simulink model "zynqRadioHWSWQPSKAD9361AD9364SL_interface"  (R2025a)
settings: Solver=FixedStepDiscrete  StartTime=0.0  StopTime=inf  RelTol=1e-3  EnableMultiTasking=on
PreLoadFcn:
  | HostIP = '192.168.3.1';
  | 
  | setTxBurstLength = 10000;
  | txtmsg = ['Zynq radio HW/SW Co-design QPSK']; % Use only printable characters
  | 
  | %------------------------------------------------------------------------------------------------------
  | 
  | if ~isequal(size(txtmsg),[1 31])
  |     error('txtmsg must contain 31 characters');
  | end
  | swTs = 0.02;
  | SamplesPerSymbol = 4;
  | Rsym = 1.92e6;
  | fs = Rsym*SamplesPerSymbol;
  | word = [txtmsg newline];
  | 
  | % The highest clock rate is 16 times the message character rate.
  | % As the message characters are fed at highest clock to FPGA
  | % repeat each character 16 times to maintain the message rate.
  | word = reshape(repmat(word,16,1),[],1);
  | repeatTimes = ceil(setTxBurstLength/length(word));
  | inpData = complex(repmat(uint8(word),repeatTimes,1));
  | inUseTxBurstLength = length(inpData);
InitFcn:
  | HostIP = '192.168.3.1';
  | 
  | setTxBurstLength = 10000;
  | txtmsg = ['Zynq radio HW/SW Co-design QPSK']; % Use only printable characters
  | 
  | %------------------------------------------------------------------------------------------------------
  | 
  | if ~isequal(size(txtmsg),[1 31])
  |     error('txtmsg must contain 31 characters');
  | end
  | swTs = 0.02;
  | SamplesPerSymbol = 4;
  | Rsym = 1.92e6;
  | fs = Rsym*SamplesPerSymbol;
  | word = [txtmsg newline];
  | 
  | % The highest clock rate is 16 times the message character rate.
  | % As the message characters are fed at highest clock to FPGA
  | % repeat each character 16 times to maintain the message rate.
  | word = reshape(repmat(word,16,1),[],1);
  | repeatTimes = ceil(setTxBurstLength/length(word));
  | inpData = complex(repmat(uint8(word),repeatTimes,1));
  | inUseTxBurstLength = length(inpData);
undefined symbols (not defined in the file or in its folder): AXI4, complex, Fs, ip, Lite
libraries: axiinterfacelib x10, zynqlib x3, xilinxsocad936xlib x2, axi_iio_lib x1, sdrzblksprivate x1
CloseFcn:
  | clear fs HostIP inpData inUseTxBurstLength ...
  |         repeatTimes Rsym SamplesPerSymbol ...
  |         setTxBurstLength swTs txtmsg word
settings Model: SimulationMode=accelerator  Creator=The MathWorks, Inc.  LastModifiedBy=The MathWorks, Inc.
settings SolverCC: AlgebraicLoopSolver=TrustRegion  PositivePriorityOrder=on  MaxZcPerStep=1.0
settings DataIOCC: ReturnWorkspaceOutputs=off
settings OptimizationCC: BlockReduction=off  ConditionallyExecuteInputs=off  EnhancedBackFolding=on  PassReuseOutputArgsAs=Individual arguments  ZeroExternalMemoryAtStartup=off  ZeroInternalMemoryAtStartup=off  MaxStackSize=64  OptimizeBlockOrder=speed  DifferentSizesBufferReuse=on  OptimizationCustomize=off  EfficientTunableParamExpr=on
settings DebuggingCC: AlgebraicLoopMsg=error  SingleTaskRateTransMsg=error  ParameterTunabilityLossMsg=error  UnconnectedInputMsg=warning  UnconnectedOutputMsg=warning  UnconnectedLineMsg=warning
settings HardwareCC: ProdBitPerPointer=32.0  ProdBitPerSizeT=32.0  ProdBitPerPtrDiffT=32.0  ProdLargestAtomicInteger=Long  ProdLargestAtomicFloat=Double  ProdWordSize=32.0  ProdLongLongMode=on  ProdHWDeviceType=ARM Compatible->ARM Cortex  TargetLargestAtomicInteger=Long  TargetLargestAtomicFloat=Double  TargetLongLongMode=on  TargetIntDivRoundTo=Zero  TargetEndianess=LittleEndian  TargetHWDeviceType=ARM Compatible->ARM Cortex
settings ModelReferenceCC: EnableRefExpFcnMdlSchedulingChecks=on  ModelReferenceNumInstancesAllowed=Single
settings SFSimCC: MATLABDynamicMemAlloc=off
settings RTWCC: SystemTargetFile=ert.tlc  HardwareBoard=Xilinx Zynq-7000 Based IIO Radio  TLCOptions="-aInlineSetEventsForThisBaseRateFcn=TLC_FALSE -aSuppressMultiTaskScheduler=TLC_FALSE  -aRateBasedStepFcn=0"  TemplateMakefile=ert_default_tmf  Toolchain=Linaro AArch32 Linux v6.3.1  GPUComputeCapability=3.5  DLArmComputeVersion=19.05  Description=Embedded Coder
settings CodeAppCC: ForceParamTrailComments=on  IgnoreCustomStorageClasses=off  OperatorAnnotations=on  SimulinkDataObjDesc=on  SFDataObjDesc=on  InsertBlockDesc=on
settings ERTTargetCC: ExtModeTransport=0.0  ExtModeStaticAlloc=off  ExtModeMexFile=ext_comm  ExtModeIntrfLevel=Level1  InlinedParameterPlacement=Hierarchical

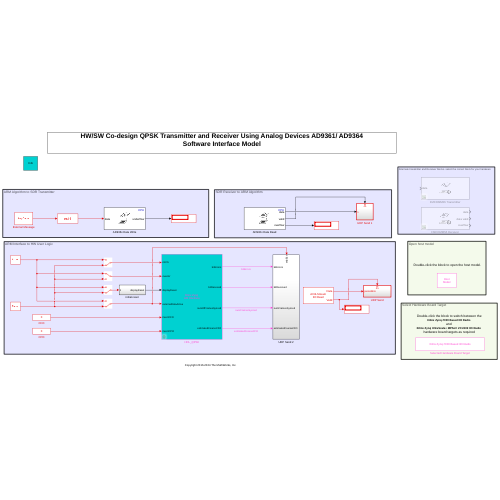
[thumbnail: Simulink's stored preview of the top-level diagram]
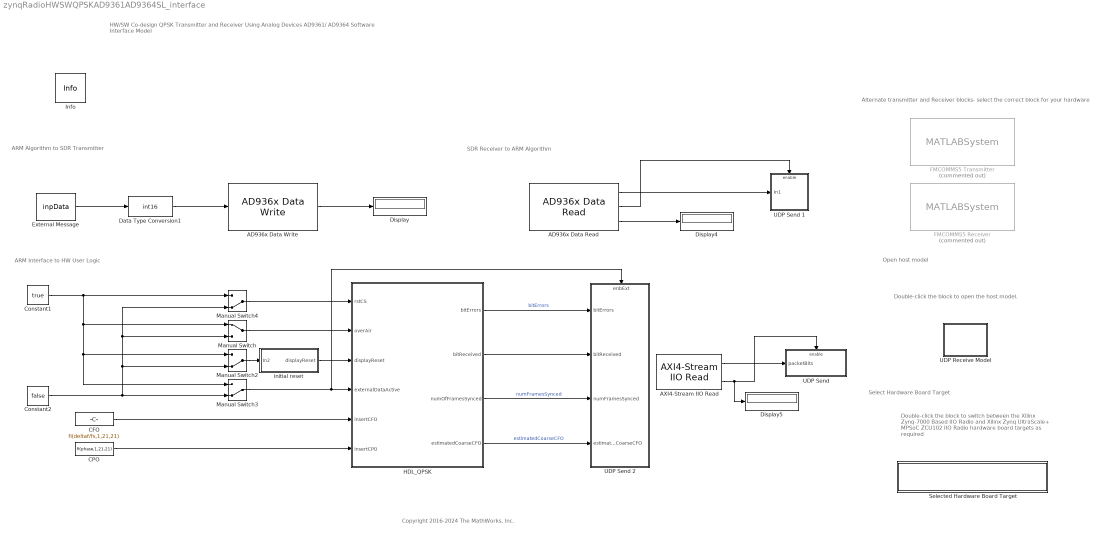
== system zynqRadioHWSWQPSKAD9361AD9364SL_interface ==
  note: ARM Interface to HW User Logic
  note: SDR Receiver to ARM Algorithm
  note: ARM Algorithm to SDR Transmitter
  note: HW/SW Co-design QPSK Transmitter and Receiver Using Analog Devices AD9361/ AD9364
      | Software Interface Model
  note: Copyright 2016-2024 The MathWorks, Inc.
  note: Alternate transmitter and Receiver blocks- select the correct block for your hardware
  note: Double-click the block to switch between the Xilinx Zynq-7000 Based IIO Radio
      | and
      | Xilinx Zynq UltraScale+ MPSoC ZCU102 IIO Radio
      | hardware board targets as required
  note: Select Hardware Board Target
  note: Double-click the block to open the host model.
  note: Open host model
  AD936x Data Read : xilinxsocad936xlib/AD936x Data Read  SimulationInput=From connected IO  IPAddress=192.168.3.2  CenterFrequencySource=Dialog  CenterFrequency=800e6  GainSource=Dialog  Gain=10  BasebandSampleRate=fs  EnableChannel1=on  EnableChannel2=off  OutputDataTypeStr=int16 (complex)  SamplesPerFrame=2048  OverflowOutputPort=on  EnableBurstMode=off  NumFramesInBurst=1  UseCustomFilter=off  filtCoefficientSize=128  filtCoefficients=round( fir1( 127, 0.75 )*2^15*10^1.2 )  filtDecimInterpFactor=4  filtGain=-12  filtPathRates=[ 737280000, 11520000, 3840000, 1920000, 960000, 240000 ]  filtRFBandwidth=18e6  filterConfigStruct=struct()  BypassUserLogic=off  EnableQuadratureCorrection=on  EnableRFDCCorrection=on  EnableBasebandDCCorrection=on  OverrideSampleTime=on  SampleTime=swTs  DataTimeout=0  BISTLoopbackMode=Disabled  BISTToneInject=Disabled  BISTSignalGen=Tone  BISTToneFreq=Fs/32  BISTToneLevel=0
      settings: LibrarySourceBlock=zynq7000zedboardlib/AD936x Data Read
  AD936x Data Write : xilinxsocad936xlib/AD936x Data Write  SimulationOutput=To connected IO  IPAddress=192.168.3.2  CenterFrequencySource=Dialog  CenterFrequency=800e6  GainSource=Dialog  Gain=0  BasebandSampleRate=fs  EnableChannel1=on  EnableChannel2=off  UnderflowOutputPort=on  UseCustomFilter=off  filtCoefficientSize=128  filtCoefficients=[-192 82 85 -215 228 -102 -110 290 -318 145 160 -426 471 -215 -238 633 -697 318 349 -923 1009 -457 -498 1309 -1423 640 693 -1812 1959 -876 -945 2458 -2647 1180 1268 -3290 3534 -1572 -1688 4375 -4698 2091 2247 -5836 6284 -2807 -3031 7918 -8588 3870 4225 -11182 12324 -5662 -6330 17255 -19735 9507 11312 -33568 43355 -25227 -42139 305542 305542 -42139 -25227 43355 -33568 11312 9507 -19735 17255 -6330 -5662 12324 -11182 4225 3870 -8588 7918 -3031 -2807 6284 -5836 2247 2091 -4698 4375 -1688 -1572 3534 -3290 1268 1180 -2647 2458 -945 -876 1959 -1812 693 640 -1423 1309 -498 -457 1009 -923 349 318 -697 633 -238 -215 471 -426 160 145 -318 290 -110 -102 228 -215 85 82 -192]  filtDecimInterpFactor=4  filtGain=-12  filtPathRates=[737280000 11520000 3840000 1920000 960000 240000]  filtRFBandwidth=18000000  filterConfigStruct=struct()  BypassUserLogic=off  DataSourceSelect=Input Port  DDSTone1Freq=5000  DDSTone2Freq=10000  DDSTone1Scale=0.5  DDSTone2Scale=0.25  DataTimeout=0  BISTLoopbackMode=Disabled  BISTToneInject=Disabled  BISTSignalGen=PRBS  BISTToneFreq=Fs/32  BISTToneLevel=0
      settings: LibrarySourceBlock=zynq7000zc706lib/AD936x Data Write
  AXI4-Stream IIO Read : axi_iio_lib/AXI4-Stream IIO Read  devName=mwipcore0:s2mm0  SamplesPerFrame=2240*2  dataTypeStr=uint32  tLastMode=auto  resetTlastMode=prebuffer  SampleTime=swTs  DataTimeout=0  uri=ip:10.0.0.200  enIO=off
  CFO : Constant  Value=fi(deltaf/fs,1,21,21)  SampleTime=swTs  mask{deltaf=0}
      mask prompts: deltaf "delta f:"
      mask Display: disp(get_param(gcb,"deltaf"));
  CPO : Constant  Value=fi(phase,1,21,21)  SampleTime=swTs  mask{phased=0}
      mask prompts: phased "phase degrees"
      mask init:
      | phase = phased/360;
      mask Display: disp(get_param(gcb,"phased"));
  Constant1 : Constant  Value=true  VectorParams1D=off  OutDataTypeStr=boolean  SampleTime=swTs
  Constant2 : Constant  Value=false  VectorParams1D=off  OutDataTypeStr=boolean  SampleTime=swTs
  Data Type Conversion1 : DataTypeConversion  OutDataTypeStr=int16  SaturateOnIntegerOverflow=off  RndMeth=Floor
  Display : Display
  Display4 : Display
  Display5 : Display
  External Message : Constant  Value=inpData  SampleTime=swTs
  FMCOMMS5 Receiver : MATLABSystem  Commented=on  System=comm.SDRRxFMCOMMS5  IPAddress=192.168.3.2  uri=ip:10.0.0.200  CenterFrequencySource=Dialog  CenterFrequency=800e6  GainSource=AGC Slow Attack  GainSourceBlock=Dialog  Gain=10  ChannelMapping=1  BasebandSampleRate=fs  OutputDataType=int16  SamplesPerFrame=2048  OverflowOutputPort=on  EnableBurstMode=off  NumFramesInBurst=1  ShowAdvancedProperties=off  UseCustomFilter=off  filtPathRates=[737280000 11520000 3840000 1920000 960000 240000]  filtCoefficients=[-192 82 85 -215 228 -102 -110 290 -318 145 160 -426 471 -215 -238 633 -697 318 349 -923 1009 -457 -498 1309 -1423 640 693 -1812 1959 -876 -945 2458 -2647 1180 1268 -3290 3534 -1572 -1688 4375 -4698 2091 2247 -5836 6284 -2807 -3031 7918 -8588 3870 4225 -11182 12324 -5662 -6330 17255 -19735 9507 11312 -33568 43355 -25227 -42139 305542 305542 -42139 -25227 43355 -33568 11312 9507 -19735 17255 -6330 -5662 12324 -11182 4225 3870 -8588 7918 -3031 -2807 6284 -5836 2247 2091 -4698 4375 -1688 -1572 3534 -3290 1268 1180 -2647 2458 -945 -876 1959 -1812 693 640 -1423 1309 -498 -457 1009 -923 349 318 -697 633 -238 -215 471 -426 160 145 -318 290 -110 -102 228 -215 85 82 -192]  filtCoefficientSize=128  filtDecimInterpFactor=4  filtGain=-12  filtRFBandwidth=18000000  filterConfigStruct=struct()  BypassUserLogic=off  EnableQuadratureCorrection=on  EnableRFDCCorrection=on  EnableBasebandDCCorrection=on  OverrideSampleTime=on  SampleTime=swTs  DataTimeout=0  ENSMPinControlMode=None  BISTLoopbackMode=Disabled  BISTToneInject=Disabled  BISTSignalGen=Tone  BISTToneFreq=Fs/32  BISTToneLevel=0
      mask Type: comm.SDRRxFMCOMMS5
  FMCOMMS5 Transmitter : MATLABSystem  Commented=on  System=comm.SDRTxFMCOMMS5  IPAddress=192.168.3.2  uri=ip:10.0.0.200  CenterFrequencySource=Dialog  CenterFrequency=800e6  GainSource=Dialog  Gain=0  ChannelMapping=1  BasebandSampleRate=fs  UnderflowOutputPort=off  ShowAdvancedProperties=off  UseCustomFilter=off  filtPathRates=[737280000 11520000 3840000 1920000 960000 240000]  filtCoefficients=[-192 82 85 -215 228 -102 -110 290 -318 145 160 -426 471 -215 -238 633 -697 318 349 -923 1009 -457 -498 1309 -1423 640 693 -1812 1959 -876 -945 2458 -2647 1180 1268 -3290 3534 -1572 -1688 4375 -4698 2091 2247 -5836 6284 -2807 -3031 7918 -8588 3870 4225 -11182 12324 -5662 -6330 17255 -19735 9507 11312 -33568 43355 -25227 -42139 305542 305542 -42139 -25227 43355 -33568 11312 9507 -19735 17255 -6330 -5662 12324 -11182 4225 3870 -8588 7918 -3031 -2807 6284 -5836 2247 2091 -4698 4375 -1688 -1572 3534 -3290 1268 1180 -2647 2458 -945 -876 1959 -1812 693 640 -1423 1309 -498 -457 1009 -923 349 318 -697 633 -238 -215 471 -426 160 145 -318 290 -110 -102 228 -215 85 82 -192]  filtCoefficientSize=128  filtDecimInterpFactor=4  filtGain=-12  filtRFBandwidth=18000000  filterConfigStruct=struct()  BypassUserLogic=off  DataSourceSelect=Input Port  DDSTone1Freq=5e3  DDSTone2Freq=10e3  DDSTone1Scale=0.5  DDSTone2Scale=0.25  DataTimeout=0  ENSMPinControlMode=None  BISTLoopbackMode=Disabled  BISTToneInject=Disabled  BISTSignalGen=Tone  BISTToneFreq=Fs/32  BISTToneLevel=0
      mask Type: comm.SDRTxFMCOMMS5
  HDL_QPSK : Subsystem
      mask Display: disp(sprintf('Xilinx Zynq \nAXI Interface'));
  Info : sdrzblksprivate/Info  SystemSampleTime=-1  VariantActivationTime=update diagram  PassThrough=off  PassThroughVariantControl=(default)  EmptyChoiceVariantControl=(default)  AllowFlexibleInterface=on  Latency=0  AutoFrameSizeCalculation=off
  Manual Switch : ManualSwitch
  Manual Switch2 : ManualSwitch  CurrentSetting=0
  Manual Switch3 : ManualSwitch  CurrentSetting=0
  Manual Switch4 : ManualSwitch  CurrentSetting=0
  Selected Hardware Board Target : Subsystem
      settings: OpenFcn=|
      | RFConfiguration = get_param(gcs, 'HardwareBoard');
      | 
      | configList = {'Xilinx Zynq-7000 Based IIO Radio', ...
      | 'Xilinx Zynq UltraScale+ MPSoC ZCU102 IIO Radio'};
      | 
      | set_param(gcs,'HardwareBoard', configList{(~strcmp(configList,RFConfiguration))});
      | set_param(gcs, 'SimulationCommand','Update');
      mask Display:
      | RFConfiguration = get_param(gcs,'HardwareBoard');
      | disp(RFConfiguration);
  UDP Receive Model : Subsystem
      settings: OpenFcn=open_system('zynqRadioHWSWQPSKAD9361AD9364SL_hostUDPReceive');
      mask Display: disp(sprintf('Host\nModel'))
  UDP Send : Subsystem
  UDP Send 1 : Subsystem
  UDP Send 2 : Subsystem
      settings: PortSchema="{\"entries\":[{\"content\":{\"sides\":[{\"content\":{\"connectorIds\":[\"In1\",\"In2\",\"In3\",\"In4\"]},\"type\":\"ConnectorPlacement.EquallySpacedRectSide\",\"uuid\":\"e0d80c2b-ac82-485a-8335-b7f1fe271b1e\"},{\"content\":{\"connectorIds\":[],\"side\":\"RIGHT\"},\"type\":\"ConnectorPlacement.EquallySpacedRectSide\",\"uuid\":\"1a9487bb-2982-46cd-8874-dab003abc3f7\"},{\"content\":{\"connectorIds\":[\"In5\"],\"side\":\"TOP\"},\"type\":\"ConnectorPlacement.EquallySpacedRectSide\",\"uuid\":\"c89cd3ff-825a-4790-95b0-6dcc2e73cf0a\"}]},\"type\":\"ConnectorPlacement.EquallySpacedConnector\",\"uuid\":\"d601894d-a5ce-417c-ae30-71bbdf43f914\"}],\"packageUris\":[\"http://schema.mathworks.com/mf0/Connector/R2020b\"],\"version\":\"1.0\"}"
  initial reset : Subsystem
  wires:
  Constant2/1 -> Manual Switch2/2, Manual Switch4/2, Manual Switch/2, Manual Switch3/2
  Manual Switch/1 -> HDL_QPSK/2(overAir)
  External Message/1 -> Data Type Conversion1/1
  HDL_QPSK/4(estimatedCoarseCFO) -> UDP Send 2/4(estimatedCoarseCFO)  "estimatedCoarseCFO"
  AD936x Data Read/2 -> UDP Send 1/Enable
  AD936x Data Read/1 -> UDP Send 1/1(In1)
  HDL_QPSK/2(bitReceived) -> UDP Send 2/2(bitReceived)
  Constant1/1 -> Manual Switch3/1, Manual Switch2/1, Manual Switch/1, Manual Switch4/1
  HDL_QPSK/3(numOfFramesSynced) -> UDP Send 2/3(numFramesSynced)  "numFramesSynced"
  AD936x Data Write/1 -> Display/1
  HDL_QPSK/1(bitErrors) -> UDP Send 2/1(bitErrors)  "bitErrors"
  Manual Switch3/1 -> HDL_QPSK/4(externalDataActive), UDP Send 2/5(enbExt)
  Manual Switch4/1 -> HDL_QPSK/1(rstCS)
  AXI4-Stream IIO Read/2 -> UDP Send/Enable, Display5/1
  AXI4-Stream IIO Read/1 -> UDP Send/1(packetBits)
  AD936x Data Read/3 -> Display4/1
  Manual Switch2/1 -> initial reset/1(In2)
  initial reset/1(displayReset) -> HDL_QPSK/3(displayReset)
  Data Type Conversion1/1 -> AD936x Data Write/1
  CFO/1 -> HDL_QPSK/5(insertCFO)
  CPO/1 -> HDL_QPSK/6(insertCPO)

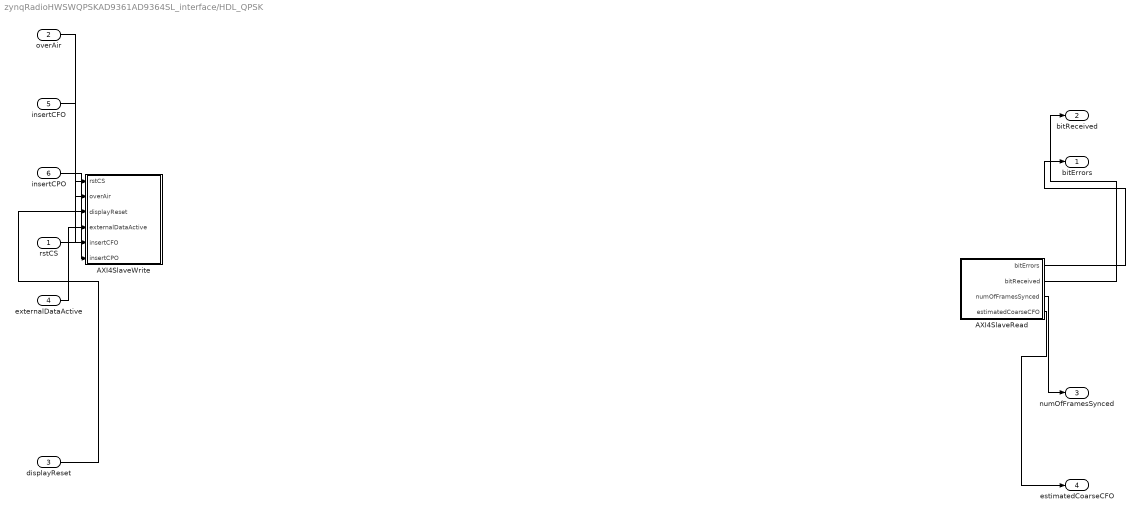
== system zynqRadioHWSWQPSKAD9361AD9364SL_interface/HDL_QPSK ==
  rstCS : Inport
  overAir : Inport  Port=2
  displayReset : Inport  Port=3
  externalDataActive : Inport  Port=4
  insertCFO : Inport  Port=5
  insertCPO : Inport  Port=6
  AXI4SlaveRead : Subsystem  Priority=10
  AXI4SlaveWrite : Subsystem  Priority=1
  bitErrors : Outport
  bitReceived : Outport  Port=2
  numOfFramesSynced : Outport  Port=3
  estimatedCoarseCFO : Outport  Port=4
  wires:
  AXI4SlaveRead/2(bitReceived) -> bitReceived/1
  AXI4SlaveRead/4(estimatedCoarseCFO) -> estimatedCoarseCFO/1
  insertCFO/1 -> AXI4SlaveWrite/5(insertCFO)
  AXI4SlaveRead/3(numOfFramesSynced) -> numOfFramesSynced/1
  AXI4SlaveRead/1(bitErrors) -> bitErrors/1
  externalDataActive/1 -> AXI4SlaveWrite/4(externalDataActive)
  displayReset/1 -> AXI4SlaveWrite/3(displayReset)
  rstCS/1 -> AXI4SlaveWrite/1(rstCS)
  insertCPO/1 -> AXI4SlaveWrite/6(insertCPO)
  overAir/1 -> AXI4SlaveWrite/2(overAir)

== system zynqRadioHWSWQPSKAD9361AD9364SL_interface/Selected Hardware Board Target ==

== system zynqRadioHWSWQPSKAD9361AD9364SL_interface/UDP Receive Model ==

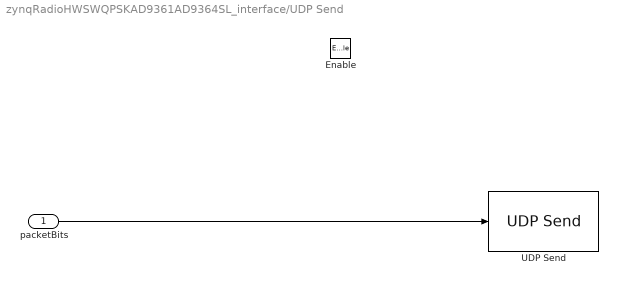
== system zynqRadioHWSWQPSKAD9361AD9364SL_interface/UDP Send ==
  packetBits : Inport
  Enable : EnablePort
  UDP Send : zynqlib/UDP Send  remoteURL=HostIP  remotePort=25000  localURL='255.255.255.255'  localPortSource=Automatically determine  localPort=-1  sendBufferSize=8192  sampletime=-1  blockPlatform=ZYNQ  separateLengthPort=0
  wires:
  packetBits/1 -> UDP Send/1

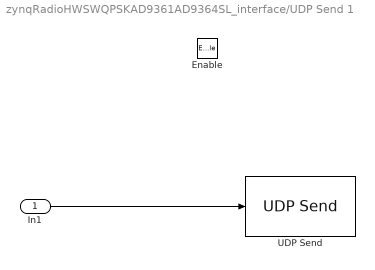
== system zynqRadioHWSWQPSKAD9361AD9364SL_interface/UDP Send 1 ==
  In1 : Inport
  Enable : EnablePort
  UDP Send : zynqlib/UDP Send  remoteURL=HostIP  remotePort=25001  localURL='255.255.255.255'  localPortSource=Automatically determine  localPort=-1  sendBufferSize=8192  sampletime=-1  blockPlatform=ZYNQ  separateLengthPort=0
  wires:
  In1/1 -> UDP Send/1

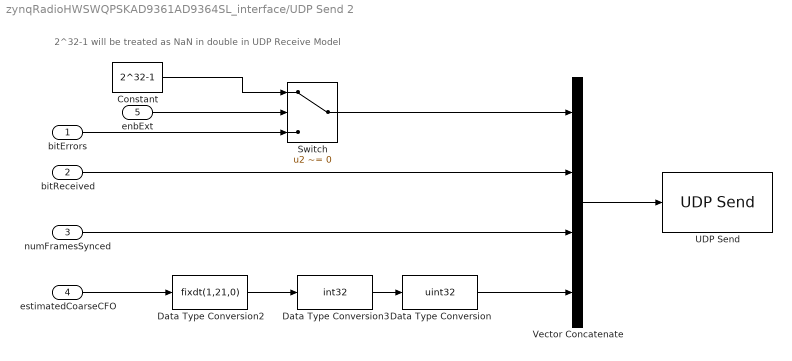
== system zynqRadioHWSWQPSKAD9361AD9364SL_interface/UDP Send 2 ==
  note: 2^32-1 will be treated as NaN in double in UDP Receive Model
  bitErrors : Inport
  bitReceived : Inport  Port=2
  numFramesSynced : Inport  Port=3
  estimatedCoarseCFO : Inport  Port=4
  enbExt : Inport  Port=5
  Constant : Constant  Value=2^32-1  OutDataTypeStr=uint32  SampleTime=-1
  Data Type Conversion : DataTypeConversion  OutDataTypeStr=uint32  ConvertRealWorld=Stored Integer (SI)  SaturateOnIntegerOverflow=off  RndMeth=Floor
  Data Type Conversion2 : DataTypeConversion  OutDataTypeStr=fixdt(1,21,0)  ConvertRealWorld=Stored Integer (SI)  SaturateOnIntegerOverflow=off  RndMeth=Floor
  Data Type Conversion3 : DataTypeConversion  OutDataTypeStr=int32  SaturateOnIntegerOverflow=off  RndMeth=Floor
  Switch : Switch  Criteria=u2 ~= 0  SaturateOnIntegerOverflow=off  InputSameDT=off
  UDP Send : zynqlib/UDP Send  remoteURL=HostIP  remotePort=25002  localURL='255.255.255.255'  localPortSource=Automatically determine  localPort=-1  sendBufferSize=8192  sampletime=-1  blockPlatform=ZYNQ  separateLengthPort=0
  Vector Concatenate : Concatenate  NumInputs=4
  wires:
  bitErrors/1 -> Switch/3
  bitReceived/1 -> Vector Concatenate/2
  numFramesSynced/1 -> Vector Concatenate/3
  estimatedCoarseCFO/1 -> Data Type Conversion2/1
  Vector Concatenate/1 -> UDP Send/1
  Data Type Conversion/1 -> Vector Concatenate/4
  Data Type Conversion2/1 -> Data Type Conversion3/1
  Data Type Conversion3/1 -> Data Type Conversion/1
  enbExt/1 -> Switch/2
  Switch/1 -> Vector Concatenate/1
  Constant/1 -> Switch/1

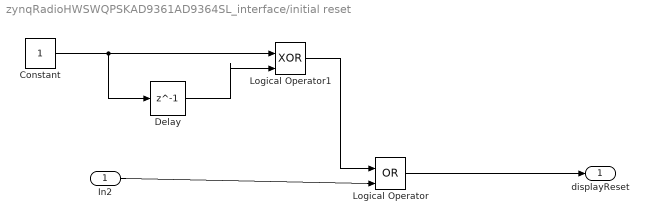
== system zynqRadioHWSWQPSKAD9361AD9364SL_interface/initial reset ==
  In2 : Inport
  Constant : Constant  OutDataTypeStr=boolean  SampleTime=-1
  Delay : Delay  DelayLength=1
  Logical Operator : Logic  Operator=OR  IconShape=distinctive  AllPortsSameDT=off  OutDataTypeStr=boolean
  Logical Operator1 : Logic  Operator=XOR  IconShape=distinctive  AllPortsSameDT=off  OutDataTypeStr=boolean
  displayReset : Outport
  wires:
  In2/1 -> Logical Operator/2
  Logical Operator1/1 -> Logical Operator/1
  Logical Operator/1 -> displayReset/1
  Constant/1 -> Delay/1, Logical Operator1/1
  Delay/1 -> Logical Operator1/2

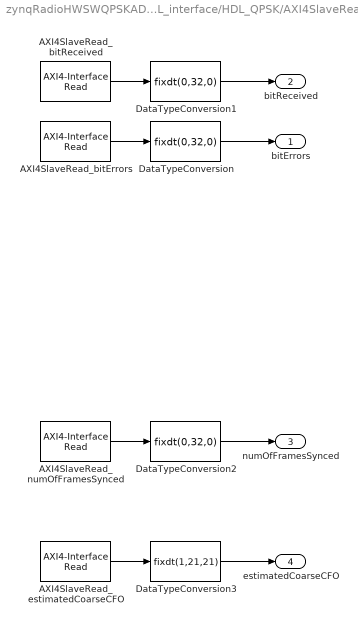
== system zynqRadioHWSWQPSKAD9361AD9364SL_interface/HDL_QPSK/AXI4SlaveRead ==
  AXI4SlaveRead_bitErrors : axiinterfacelib/AXI4-Interface Read  Priority=3  AXIInterfaceType=AXI4-Lite  DeviceName=/dev/mwipcore  RegisterOffset=hex2dec('118')  DataLength=1  DataType=uint32  SampleTime=-1  blockPlatform=ZYNQ  SimulateUsing=Interpreted Execution
  AXI4SlaveRead_bitReceived : axiinterfacelib/AXI4-Interface Read  Priority=4  AXIInterfaceType=AXI4-Lite  DeviceName=/dev/mwipcore  RegisterOffset=hex2dec('11C')  DataLength=1  DataType=uint32  SampleTime=-1  blockPlatform=ZYNQ  SimulateUsing=Interpreted Execution
  AXI4SlaveRead_estimatedCoarseCFO : axiinterfacelib/AXI4-Interface Read  Priority=6  AXIInterfaceType=AXI4-Lite  DeviceName=/dev/mwipcore  RegisterOffset=hex2dec('124')  DataLength=1  DataType=uint32  SampleTime=-1  blockPlatform=ZYNQ  SimulateUsing=Interpreted Execution
  AXI4SlaveRead_numOfFramesSynced : axiinterfacelib/AXI4-Interface Read  Priority=5  AXIInterfaceType=AXI4-Lite  DeviceName=/dev/mwipcore  RegisterOffset=hex2dec('120')  DataLength=1  DataType=uint32  SampleTime=-1  blockPlatform=ZYNQ  SimulateUsing=Interpreted Execution
  DataTypeConversion : DataTypeConversion  OutDataTypeStr=fixdt(0,32,0)  ConvertRealWorld=Stored Integer (SI)  SaturateOnIntegerOverflow=off  RndMeth=Floor
  DataTypeConversion1 : DataTypeConversion  OutDataTypeStr=fixdt(0,32,0)  ConvertRealWorld=Stored Integer (SI)  SaturateOnIntegerOverflow=off  RndMeth=Floor
  DataTypeConversion2 : DataTypeConversion  OutDataTypeStr=fixdt(0,32,0)  ConvertRealWorld=Stored Integer (SI)  SaturateOnIntegerOverflow=off  RndMeth=Floor
  DataTypeConversion3 : DataTypeConversion  OutDataTypeStr=fixdt(1,21,21)  ConvertRealWorld=Stored Integer (SI)  SaturateOnIntegerOverflow=off  RndMeth=Floor
  bitErrors : Outport
  bitReceived : Outport  Port=2
  numOfFramesSynced : Outport  Port=3
  estimatedCoarseCFO : Outport  Port=4
  wires:
  AXI4SlaveRead_bitReceived/1 -> DataTypeConversion1/1
  AXI4SlaveRead_numOfFramesSynced/1 -> DataTypeConversion2/1
  DataTypeConversion2/1 -> numOfFramesSynced/1
  DataTypeConversion/1 -> bitErrors/1
  AXI4SlaveRead_bitErrors/1 -> DataTypeConversion/1
  DataTypeConversion3/1 -> estimatedCoarseCFO/1
  DataTypeConversion1/1 -> bitReceived/1
  AXI4SlaveRead_estimatedCoarseCFO/1 -> DataTypeConversion3/1

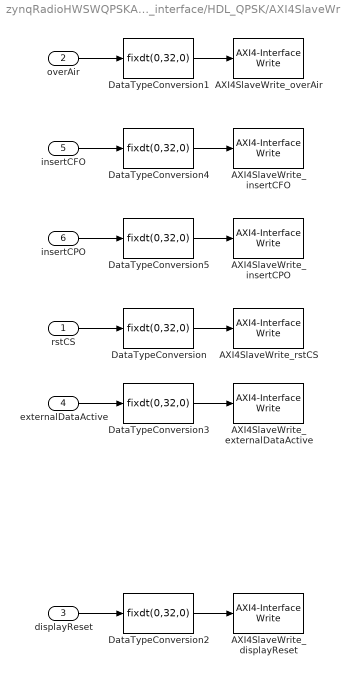
== system zynqRadioHWSWQPSKAD9361AD9364SL_interface/HDL_QPSK/AXI4SlaveWrite ==
  rstCS : Inport
  overAir : Inport  Port=2
  displayReset : Inport  Port=3
  externalDataActive : Inport  Port=4
  insertCFO : Inport  Port=5
  insertCPO : Inport  Port=6
  AXI4SlaveWrite_displayReset : axiinterfacelib/AXI4-Interface Write  Priority=4  AXIInterfaceType=AXI4-Lite  DeviceName=/dev/mwipcore  RegisterOffset=hex2dec('108')  blockPlatform=ZYNQ  SimulateUsing=Interpreted execution
  AXI4SlaveWrite_externalDataActive : axiinterfacelib/AXI4-Interface Write  Priority=5  AXIInterfaceType=AXI4-Lite  DeviceName=/dev/mwipcore  RegisterOffset=hex2dec('10C')  blockPlatform=ZYNQ  SimulateUsing=Interpreted execution
  AXI4SlaveWrite_insertCFO : axiinterfacelib/AXI4-Interface Write  Priority=6  AXIInterfaceType=AXI4-Lite  DeviceName=/dev/mwipcore  RegisterOffset=hex2dec('110')  blockPlatform=ZYNQ  SimulateUsing=Interpreted execution
  AXI4SlaveWrite_insertCPO : axiinterfacelib/AXI4-Interface Write  Priority=7  AXIInterfaceType=AXI4-Lite  DeviceName=/dev/mwipcore  RegisterOffset=hex2dec('114')  blockPlatform=ZYNQ  SimulateUsing=Interpreted execution
  AXI4SlaveWrite_overAir : axiinterfacelib/AXI4-Interface Write  Priority=3  AXIInterfaceType=AXI4-Lite  DeviceName=/dev/mwipcore  RegisterOffset=hex2dec('104')  blockPlatform=ZYNQ  SimulateUsing=Interpreted execution
  AXI4SlaveWrite_rstCS : axiinterfacelib/AXI4-Interface Write  Priority=2  AXIInterfaceType=AXI4-Lite  DeviceName=/dev/mwipcore  RegisterOffset=hex2dec('100')  blockPlatform=ZYNQ  SimulateUsing=Interpreted execution
  DataTypeConversion{,1..5} (6 alike) : DataTypeConversion  OutDataTypeStr=fixdt(0,32,0)  ConvertRealWorld=Stored Integer (SI)  SaturateOnIntegerOverflow=off  RndMeth=Floor
  wires:
  externalDataActive/1 -> DataTypeConversion3/1
  DataTypeConversion/1 -> AXI4SlaveWrite_rstCS/1
  DataTypeConversion2/1 -> AXI4SlaveWrite_displayReset/1
  insertCFO/1 -> DataTypeConversion4/1
  DataTypeConversion4/1 -> AXI4SlaveWrite_insertCFO/1
  rstCS/1 -> DataTypeConversion/1
  displayReset/1 -> DataTypeConversion2/1
  DataTypeConversion3/1 -> AXI4SlaveWrite_externalDataActive/1
  DataTypeConversion5/1 -> AXI4SlaveWrite_insertCPO/1
  overAir/1 -> DataTypeConversion1/1
  insertCPO/1 -> DataTypeConversion5/1
  DataTypeConversion1/1 -> AXI4SlaveWrite_overAir/1
